simulink model "PD_Ops"  (R2017a)
settings: Solver=ode15s  StartTime=0.0  StopTime=10  RelTol=1e-4
values from neighbouring files (symbols this model uses):
  Kd = 50*eye(7)    [forwardDynamics.m]
  Kp = 500*eye(7)    [forwardDynamics.m]
  m = num2cell(m)    [CoriolisTerm.m]    (also in GravityTerm.m; InvDynNum.m; InverseDynamics.m = [mA mB mC mD mE mF mG]; MassMatrix.m)
libraries: mblibv1 x36, simulink x2
(part 1 of 2)
settings Model: Creator=litianyi  LastModifiedBy=nathaliemajcherczyk
settings SolverCC: ZeroCrossControl=DisableAll

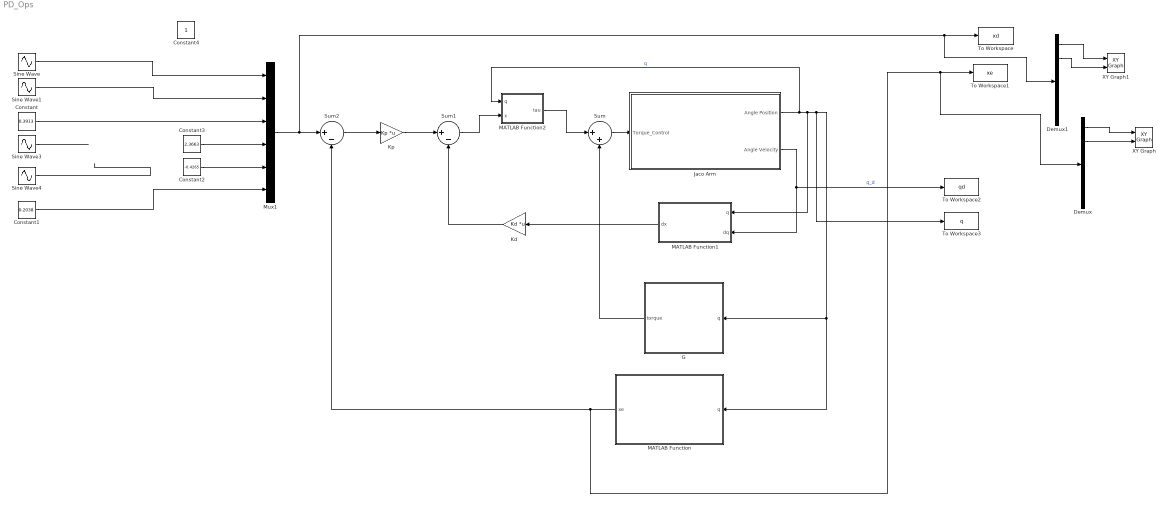
== system PD_Ops ==
  Constant : Constant  Value=0.3913  VectorParams1D=off
  Constant1 : Constant  Value=0.2038  VectorParams1D=off
  Constant2 : Constant  Value=-0.4265  VectorParams1D=off
  Constant3 : Constant  Value=2.3663  VectorParams1D=off
  Constant4 : Constant  VectorParams1D=off
  Demux : Demux  Outputs=6
  Demux1 : Demux  Outputs=6
  G : MATLAB Function  TreatAsAtomicUnit=on
  "Jaco Arm " : Subsystem
  Kd : Gain  Gain=Kd  Multiplication=Matrix(K*u)
  Kp : Gain  Gain=Kp  Multiplication=Matrix(K*u)
  MATLAB Function : MATLAB Function  TreatAsAtomicUnit=on
  MATLAB Function1 : MATLAB Function  TreatAsAtomicUnit=on
  MATLAB Function2 : MATLAB Function  TreatAsAtomicUnit=on
  Mux1 : Mux  Inputs=6
  Sine Wave : Sin  Amplitude=0.2  Bias=0.0075  Phase=pi/2  SampleTime=0
  Sine Wave1 : Sin  Amplitude=0.2  Bias=-0.0204  SampleTime=0
  Sine Wave3 : Sin  Amplitude=10  Phase=pi  SampleTime=0
  Sine Wave4 : Sin  Amplitude=10  Bias=-10  Phase=pi/2  SampleTime=0
  Sum : Sum  Inputs=|++
  Sum1 : Sum  Inputs=|+-
  Sum2 : Sum  Inputs=|+-
  To Workspace : ToWorkspace  VariableName=xd  SaveFormat=Timeseries  SampleTime=-1
  To Workspace1 : ToWorkspace  VariableName=xe  SaveFormat=Timeseries  SampleTime=-1
  To Workspace2 : ToWorkspace  VariableName=qd  SaveFormat=Timeseries  SampleTime=-1
  To Workspace3 : ToWorkspace  VariableName=q  SaveFormat=Timeseries  SampleTime=-1
  XY Graph : simulink/Sinks/XY Graph  xmin=-1  xmax=1  ymin=-1  ymax=1  st=-1
  XY Graph1 : simulink/Sinks/XY Graph  xmin=-1  xmax=1  ymin=-1  ymax=1  st=-1
  wires:
  Kd/1 -> Sum1/2
  "Jaco Arm "/2(Angle Velocity) -> To Workspace2/1, MATLAB Function1/2(dq)  "q_d"
  Kp/1 -> Sum1/1
  "Jaco Arm "/1("Angle Position ") -> MATLAB Function2/1(q), MATLAB Function1/1(q), To Workspace3/1, G/1(q), MATLAB Function/1(q)  "q"
  Sum/1 -> "Jaco Arm "/1("Torque_Control ")
  Sum2/1 -> Kp/1
  G/1(torque) -> Sum/2
  Constant/1 -> Mux1/3
  Constant1/1 -> Mux1/6
  MATLAB Function1/1(dx) -> Kd/1
  MATLAB Function2/1(tau) -> Sum/1
  MATLAB Function/1(xe) -> Demux/1, To Workspace1/1, Sum2/2
  Sum1/1 -> MATLAB Function2/2(x)
  Sine Wave4/1 -> ?
  Sine Wave3/1 -> ?
  Mux1/1 -> Demux1/1, To Workspace/1, Sum2/1
  Demux/1 -> XY Graph/1
  Demux/2 -> XY Graph/2
  Demux1/1 -> XY Graph1/1
  Demux1/2 -> XY Graph1/2
  Sine Wave1/1 -> Mux1/2
  Sine Wave/1 -> Mux1/1
  Constant3/1 -> Mux1/4
  Constant2/1 -> Mux1/5

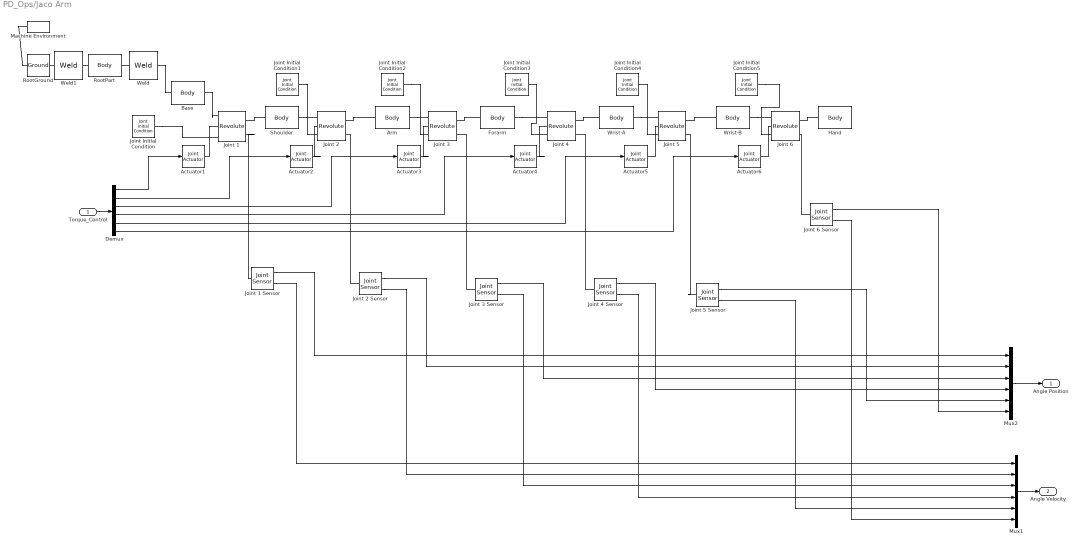
== system PD_Ops/Jaco Arm  ==
  "Torque_Control " : Inport
  Actuator{1..6} (6 alike) : mblibv1/Sensors &  Actuators/Joint Actuator  UpdateFromCAD=off  PhysicalDomain=Mechanical  PortType=blob  ActuationStyle=Force  AngleUnits=deg  ArcVelocityUnits=deg/s  ArcAccelerationUnits=deg/s^2  CoordPositionUnits=m  VelocityUnits=m/s  AccelerationUnits=m/s^2  ForceUnits=N  TorqueUnits=N-m  ActiveIO=on  Width=1  DialogClass=MechanicalActuatorBlock  Primitive=R1  ReferenceFrame=Absolute (World)
      settings: SourceProductName=Simscape Multibody  SourceProductBaseCode=MS
  Arm : mblibv1/Bodies/Body  LConnTagsString=CS2  RConnTagsString=CS3  UpdateFromCAD=on  DialogClass=MechanicalBodyBlock  Mass=1.056  MassUnits=kg  InertiaUnits=kg*m^2  Inertia=[0.0375645,-1.33324e-07,0.000108785;-1.33324e-07,0.0372402,-2.39225e-07;0.000108785,-2.39225e-07,0.00059301]  Shape=Cylinder  ShapeDims=[1 1]  ShapeUnits=m  ShapeUse=false  Density=1  DensityUnits=kg/m^3  DensityUse=false  GraphicsMode=GFXFILE  GraphicsFileName=Jaco_3_7 - arm_ass-1.STL  BodyColorSelMode=COLORPALETTE  BodyColor=[0.752941;0.752941;0.752941]  AttachedToCS=CS1  CG=Right$CG$[0.10282 0.0944444 0.508793]$WORLD$WORLD$m$[0.695251 0.715707 -0.0662524;0.718767 -0.692291 0.0640847;0 -0.092175 -0.995743]$3x3 Transform$rad$WORLD$false$none  WorkingFrames=Right$CS1$[-0.183907 0.105598 0.903425]$WORLD$WORLD$m$[0.695251 0.715707 -0.0662524;0.718767 -0.692291 0.0640847;0 -0.092175 -0.995743]$3x3 Transform$rad$WORLD$false$none#Left$CS2$[0.0767642 0.095252 0.300589]$WORLD$WORLD$m$[1 0 0;0 1 0;0 0 1]$3x3 Transform$rad$WORLD$true$none#Right$CS3$[0.10358 0.0686179 0.708843]$WORLD$WORLD$m$[1 0 0;0 1 0;0 0 1]$3x3 Transform$rad$WORLD$true$none  CGPos=[0.10282 0.0944444 0.508793]  CGRot=[0.695251 0.715707 -0.0662524;0.718767 -0.692291 0.0640847;0 -0.092175 -0.995743]  CS0Pos=[]  CS0Rot=[]  CS1Pos=[-0.183907 0.105598 0.903425]  CS1Rot=[0.695251 0.715707 -0.0662524;0.718767 -0.692291 0.0640847;0 -0.092175 -0.995743]  CS2Pos=[0.0767642 0.095252 0.300589]  CS2Rot=[1 0 0;0 1 0;0 0 1]  CS3Pos=[0.10358 0.0686179 0.708843]  CS3Rot=[1 0 0;0 1 0;0 0 1]  CS4Pos=[]  CS4Rot=[]  CS5Pos=[]  CS5Rot=[]  CS6Pos=[]  CS6Rot=[]  CS7Pos=[]  CS7Rot=[]  CS8Pos=[]  CS8Rot=[]  CS9Pos=[]  CS9Rot=[]  CS10Pos=[]  CS10Rot=[]  CS11Pos=[]  CS11Rot=[]  CS12Pos=[]  CS12Rot=[]  CS13Pos=[]  CS13Rot=[]  CS14Pos=[]  CS14Rot=[]  CS15Pos=[]  CS15Rot=[]  CS16Pos=[]  CS16Rot=[]  CS17Pos=[]  CS17Rot=[]  CS18Pos=[]  CS18Rot=[]  CS19Pos=[]  CS19Rot=[]  CS20Pos=[]  CS20Rot=[]
      settings: SourceProductName=Simscape Multibody  SourceProductBaseCode=MS
  Base : mblibv1/Bodies/Body  LConnTagsString=CS2  RConnTagsString=CS3  UpdateFromCAD=on  DialogClass=MechanicalBodyBlock  Mass=0.570939  MassUnits=kg  InertiaUnits=kg*m^2  Inertia=[0.00175947,1.92772e-07,-3.1782e-05;1.92772e-07,0.00176256,-3.18122e-05;-3.1782e-05,-3.18122e-05,0.000478232]  Shape=Cylinder  ShapeDims=[1 1]  ShapeUnits=m  ShapeUse=false  Density=1  DensityUnits=kg/m^3  DensityUse=false  GraphicsMode=GFXFILE  GraphicsFileName=Jaco_3_7 - base_ass-1.STL  BodyColorSelMode=COLORPALETTE  BodyColor=[0.752941;0.752941;0.752941]  AttachedToCS=CS1  CG=Right$CG$[0.0747134 0.093124 0.128067]$WORLD$WORLD$m$[1 0 0;0 1 0;0 0 1]$3x3 Transform$rad$WORLD$false$none  WorkingFrames=Right$CS1$[0.106448 0.0299726 -0.0762042]$WORLD$WORLD$m$[1 0 0;0 1 0;0 0 1]$3x3 Transform$rad$WORLD$false$none#Left$CS2$[0.0747134 0.093124 0.128067]$WORLD$WORLD$m$[1 0 0;0 1 0;0 0 1]$3x3 Transform$rad$WORLD$true$none#Right$CS3$[0.0753736 0.0938145 0.182089]$WORLD$WORLD$m$[1 0 0;0 1 0;0 0 1]$3x3 Transform$rad$WORLD$true$none  CGPos=[0.0747134 0.093124 0.128067]  CGRot=[1 0 0;0 1 0;0 0 1]  CS0Pos=[]  CS0Rot=[]  CS1Pos=[0.106448 0.0299726 -0.0762042]  CS1Rot=[1 0 0;0 1 0;0 0 1]  CS2Pos=[0.0747134 0.093124 0.128067]  CS2Rot=[1 0 0;0 1 0;0 0 1]  CS3Pos=[0.0753736 0.0938145 0.182089]  CS3Rot=[1 0 0;0 1 0;0 0 1]  CS4Pos=[]  CS4Rot=[]  CS5Pos=[]  CS5Rot=[]  CS6Pos=[]  CS6Rot=[]  CS7Pos=[]  CS7Rot=[]  CS8Pos=[]  CS8Rot=[]  CS9Pos=[]  CS9Rot=[]  CS10Pos=[]  CS10Rot=[]  CS11Pos=[]  CS11Rot=[]  CS12Pos=[]  CS12Rot=[]  CS13Pos=[]  CS13Rot=[]  CS14Pos=[]  CS14Rot=[]  CS15Pos=[]  CS15Rot=[]  CS16Pos=[]  CS16Rot=[]  CS17Pos=[]  CS17Rot=[]  CS18Pos=[]  CS18Rot=[]  CS19Pos=[]  CS19Rot=[]  CS20Pos=[]  CS20Rot=[]
      settings: SourceProductName=Simscape Multibody  SourceProductBaseCode=MS
  Demux : Demux  Outputs=6
  Forarm : mblibv1/Bodies/Body  LConnTagsString=CS2  RConnTagsString=CS3  UpdateFromCAD=on  DialogClass=MechanicalBodyBlock  Mass=0.735414  MassUnits=kg  InertiaUnits=kg*m^2  Inertia=[0.00626271,-0.000115651,1.81814e-08;-0.000115651,0.000377159,4.13244e-07;1.81814e-08,4.13244e-07,0.00610747]  Shape=Cylinder  ShapeDims=[1 1]  ShapeUnits=m  ShapeUse=false  Density=1  DensityUnits=kg/m^3  DensityUse=false  GraphicsMode=GFXFILE  GraphicsFileName=Jaco_3_7 - forarm_ass-1.STL  BodyColorSelMode=COLORPALETTE  BodyColor=[0.752941;0.752941;0.752941]  AttachedToCS=CS1  CG=Right$CG$[0.142291 0.0111153 0.740623]$WORLD$WORLD$m$[0.695251 0.650811 0.305076;0.718767 -0.629518 -0.295094;0 0.424443 -0.905455]$3x3 Transform$rad$WORLD$false$none  WorkingFrames=Right$CS1$[-0.0310579 0.0970807 0.899014]$WORLD$WORLD$m$[0.695251 0.650811 0.305076;0.718767 -0.629518 -0.295094;0 0.424443 -0.905455]$3x3 Transform$rad$WORLD$false$none#Left$CS2$[0.10358 0.0686179 0.708843]$WORLD$WORLD$m$[1 0 0;0 1 0;0 0 1]$3x3 Transform$rad$WORLD$true$none#Right$CS3$[0.230802 -0.0700932 0.796915]$WORLD$WORLD$m$[1 0 0;0 1 0;0 0 1]$3x3 Transform$rad$WORLD$true$none  CGPos=[0.142291 0.0111153 0.740623]  CGRot=[0.695251 0.650811 0.305076;0.718767 -0.629518 -0.295094;0 0.424443 -0.905455]  CS0Pos=[]  CS0Rot=[]  CS1Pos=[-0.0310579 0.0970807 0.899014]  CS1Rot=[0.695251 0.650811 0.305076;0.718767 -0.629518 -0.295094;0 0.424443 -0.905455]  CS2Pos=[0.10358 0.0686179 0.708843]  CS2Rot=[1 0 0;0 1 0;0 0 1]  CS3Pos=[0.230802 -0.0700932 0.796915]  CS3Rot=[1 0 0;0 1 0;0 0 1]  CS4Pos=[]  CS4Rot=[]  CS5Pos=[]  CS5Rot=[]  CS6Pos=[]  CS6Rot=[]  CS7Pos=[]  CS7Rot=[]  CS8Pos=[]  CS8Rot=[]  CS9Pos=[]  CS9Rot=[]  CS10Pos=[]  CS10Rot=[]  CS11Pos=[]  CS11Rot=[]  CS12Pos=[]  CS12Rot=[]  CS13Pos=[]  CS13Rot=[]  CS14Pos=[]  CS14Rot=[]  CS15Pos=[]  CS15Rot=[]  CS16Pos=[]  CS16Rot=[]  CS17Pos=[]  CS17Rot=[]  CS18Pos=[]  CS18Rot=[]  CS19Pos=[]  CS19Rot=[]  CS20Pos=[]  CS20Rot=[]
      settings: SourceProductName=Simscape Multibody  SourceProductBaseCode=MS
  Hand : mblibv1/Bodies/Body  LConnTagsString=CS2  UpdateFromCAD=on  DialogClass=MechanicalBodyBlock  Mass=0.395999  MassUnits=kg  InertiaUnits=kg*m^2  Inertia=[0.00124769,-0.000197969,-5.51354e-06;-0.000197969,0.000409818,-2.12169e-05;-5.51354e-06,-2.12169e-05,0.00139509]  Shape=Cylinder  ShapeDims=[1 1]  ShapeUnits=m  ShapeUse=false  Density=1  DensityUnits=kg/m^3  DensityUse=false  GraphicsMode=GFXFILE  GraphicsFileName=Jaco_3_7 - Hand_ass-1.STL  BodyColorSelMode=COLORPALETTE  BodyColor=[0.752941;0.752941;0.752941]  AttachedToCS=CS1  CG=Right$CG$[0.35442 -0.232757 0.799495]$WORLD$WORLD$m$[-0.439555 0.858973 -0.262597;-0.828489 -0.500657 -0.250895;-0.346983 0.107276 0.931716]$3x3 Transform$rad$WORLD$false$none  WorkingFrames=Right$CS1$[0.362295 -0.115327 0.65151]$WORLD$WORLD$m$[-0.439555 0.858973 -0.262597;-0.828489 -0.500657 -0.250895;-0.346983 0.107276 0.931716]$3x3 Transform$rad$WORLD$false$none#Left$CS2$[0.306767 -0.196631 0.795235]$WORLD$WORLD$m$[1 0 0;0 1 0;0 0 1]$3x3 Transform$rad$WORLD$true$none  CGPos=[0.35442 -0.232757 0.799495]  CGRot=[-0.439555 0.858973 -0.262597;-0.828489 -0.500657 -0.250895;-0.346983 0.107276 0.931716]  CS0Pos=[]  CS0Rot=[]  CS1Pos=[0.362295 -0.115327 0.65151]  CS1Rot=[-0.439555 0.858973 -0.262597;-0.828489 -0.500657 -0.250895;-0.346983 0.107276 0.931716]  CS2Pos=[0.306767 -0.196631 0.795235]  CS2Rot=[1 0 0;0 1 0;0 0 1]  CS3Pos=[]  CS3Rot=[]  CS4Pos=[]  CS4Rot=[]  CS5Pos=[]  CS5Rot=[]  CS6Pos=[]  CS6Rot=[]  CS7Pos=[]  CS7Rot=[]  CS8Pos=[]  CS8Rot=[]  CS9Pos=[]  CS9Rot=[]  CS10Pos=[]  CS10Rot=[]  CS11Pos=[]  CS11Rot=[]  CS12Pos=[]  CS12Rot=[]  CS13Pos=[]  CS13Rot=[]  CS14Pos=[]  CS14Rot=[]  CS15Pos=[]  CS15Rot=[]  CS16Pos=[]  CS16Rot=[]  CS17Pos=[]  CS17Rot=[]  CS18Pos=[]  CS18Rot=[]  CS19Pos=[]  CS19Rot=[]  CS20Pos=[]  CS20Rot=[]
      settings: SourceProductName=Simscape Multibody  SourceProductBaseCode=MS
  Joint 1 : mblibv1/Joints/Revolute  LConnTagsString=__newl0|SA1|SA2  RConnTagsString=__newr0|SA1  UpdateFromCAD=on  NumSAPorts=3  CutJoint=off  MarkAsCut=off  Primitives=prismatic  PrimitiveProps=R1$World$[0,0,1]$revolute  DialogClass=JointBlock  R1Axis=[0,0,1]
      settings: SourceProductName=Simscape Multibody  SourceProductBaseCode=MS
  Joint 1 Sensor : mblibv1/Sensors &  Actuators/Joint Sensor  UpdateFromCAD=off  PhysicalDomain=Mechanical  PortType=blob  Muxed=off  Pose=off  Angle=on  AngleUnits=rad  ArcVelocity=on  ArcVelocityUnits=rad/s  ArcAcceleration=off  ArcAccelerationUnits=deg/s^2  CoordPosition=on  CoordPositionUnits=m  Velocity=off  VelocityUnits=m/s  Acceleration=off  AccelerationUnits=m/s^2  Quaternion=on  QuaternionDT=off  QuaternionDDT=off  QuaternionUnits=off  OutputVector=[1]  ActiveIO=on  Width=2  DialogClass=MechanicalSensorBlock  Primitive=R1  Force=off  ForceUnits=N  Torque=off  TorqueUnits=N*m  ReferenceFrame=Absolute (World)  ReactionSensedSide=Base  ReactionReferenceFrame=Absolute (World)  ReactionForce=off  ReactionForceUnits=N  ReactionMoment=off  ReactionMomentUnits=N*m
      settings: SourceProductName=Simscape Multibody  SourceProductBaseCode=MS
  Joint 2 : mblibv1/Joints/Revolute  LConnTagsString=__newl0|SA1|SA2  RConnTagsString=__newr0|SA1  UpdateFromCAD=on  NumSAPorts=3  CutJoint=off  MarkAsCut=off  Primitives=prismatic  PrimitiveProps=R1$World$[0.695251,0.718767,0]$revolute  DialogClass=JointBlock  R1Axis=[0.695251,0.718767,0]
      settings: SourceProductName=Simscape Multibody  SourceProductBaseCode=MS
  Joint 2 Sensor : mblibv1/Sensors &  Actuators/Joint Sensor  UpdateFromCAD=off  PhysicalDomain=Mechanical  PortType=blob  Muxed=off  Pose=off  Angle=on  AngleUnits=rad  ArcVelocity=on  ArcVelocityUnits=rad/s  ArcAcceleration=off  ArcAccelerationUnits=deg/s^2  CoordPosition=on  CoordPositionUnits=m  Velocity=off  VelocityUnits=m/s  Acceleration=off  AccelerationUnits=m/s^2  Quaternion=on  QuaternionDT=off  QuaternionDDT=off  QuaternionUnits=off  OutputVector=[1]  ActiveIO=on  Width=2  DialogClass=MechanicalSensorBlock  Primitive=R1  Force=off  ForceUnits=N  Torque=off  TorqueUnits=N*m  ReferenceFrame=Absolute (World)  ReactionSensedSide=Base  ReactionReferenceFrame=Absolute (World)  ReactionForce=off  ReactionForceUnits=N  ReactionMoment=off  ReactionMomentUnits=N*m
      settings: SourceProductName=Simscape Multibody  SourceProductBaseCode=MS
  Joint 3 : mblibv1/Joints/Revolute  LConnTagsString=__newl0|SA1|SA2  RConnTagsString=__newr0|SA1  UpdateFromCAD=on  NumSAPorts=3  CutJoint=off  MarkAsCut=off  Primitives=prismatic  PrimitiveProps=R1$World$[-0.695251,-0.718767,0]$revolute  DialogClass=JointBlock  R1Axis=[-0.695251,-0.718767,0]
      settings: SourceProductName=Simscape Multibody  SourceProductBaseCode=MS
  Joint 3 Sensor : mblibv1/Sensors &  Actuators/Joint Sensor  UpdateFromCAD=off  PhysicalDomain=Mechanical  PortType=blob  Muxed=off  Pose=off  Angle=on  AngleUnits=rad  ArcVelocity=on  ArcVelocityUnits=rad/s  ArcAcceleration=off  ArcAccelerationUnits=deg/s^2  CoordPosition=on  CoordPositionUnits=m  Velocity=off  VelocityUnits=m/s  Acceleration=off  AccelerationUnits=m/s^2  Quaternion=on  QuaternionDT=off  QuaternionDDT=off  QuaternionUnits=off  OutputVector=[1]  ActiveIO=on  Width=2  DialogClass=MechanicalSensorBlock  Primitive=R1  Force=off  ForceUnits=N  Torque=off  TorqueUnits=N*m  ReferenceFrame=Absolute (World)  ReactionSensedSide=Base  ReactionReferenceFrame=Absolute (World)  ReactionForce=off  ReactionForceUnits=N  ReactionMoment=off  ReactionMomentUnits=N*m
      settings: SourceProductName=Simscape Multibody  SourceProductBaseCode=MS
  Joint 4 : mblibv1/Joints/Revolute  LConnTagsString=__newl0|SA1|SA2  RConnTagsString=__newr0|SA1  UpdateFromCAD=on  NumSAPorts=3  CutJoint=off  MarkAsCut=off  Primitives=prismatic  PrimitiveProps=R1$World$[0.650811,-0.629518,0.424443]$revolute  DialogClass=JointBlock  R1Axis=[0.650811,-0.629518,0.424443]
      settings: SourceProductName=Simscape Multibody  SourceProductBaseCode=MS
  Joint 4 Sensor : mblibv1/Sensors &  Actuators/Joint Sensor  UpdateFromCAD=off  PhysicalDomain=Mechanical  PortType=blob  Muxed=off  Pose=off  Angle=on  AngleUnits=rad  ArcVelocity=on  ArcVelocityUnits=rad/s  ArcAcceleration=off  ArcAccelerationUnits=deg/s^2  CoordPosition=on  CoordPositionUnits=m  Velocity=off  VelocityUnits=m/s  Acceleration=off  AccelerationUnits=m/s^2  Quaternion=on  QuaternionDT=off  QuaternionDDT=off  QuaternionUnits=off  OutputVector=[1]  ActiveIO=on  Width=2  DialogClass=MechanicalSensorBlock  Primitive=R1  Force=off  ForceUnits=N  Torque=off  TorqueUnits=N*m  ReferenceFrame=Absolute (World)  ReactionSensedSide=Base  ReactionReferenceFrame=Absolute (World)  ReactionForce=off  ReactionForceUnits=N  ReactionMoment=off  ReactionMomentUnits=N*m
      settings: SourceProductName=Simscape Multibody  SourceProductBaseCode=MS
  Joint 5 : mblibv1/Joints/Revolute  LConnTagsString=__newl0|SA1|SA2  RConnTagsString=__newr0|SA1  UpdateFromCAD=on  NumSAPorts=3  CutJoint=off  MarkAsCut=off  Primitives=prismatic  PrimitiveProps=R1$World$[0.15169,-0.946456,-0.284976]$revolute  DialogClass=JointBlock  R1Axis=[0.15169,-0.946456,-0.284976]
      settings: SourceProductName=Simscape Multibody  SourceProductBaseCode=MS
  Joint 5 Sensor : mblibv1/Sensors &  Actuators/Joint Sensor  UpdateFromCAD=off  PhysicalDomain=Mechanical  PortType=blob  Muxed=off  Pose=off  Angle=on  AngleUnits=rad  ArcVelocity=on  ArcVelocityUnits=rad/s  ArcAcceleration=off  ArcAccelerationUnits=deg/s^2  CoordPosition=on  CoordPositionUnits=m  Velocity=off  VelocityUnits=m/s  Acceleration=off  AccelerationUnits=m/s^2  Quaternion=on  QuaternionDT=off  QuaternionDDT=off  QuaternionUnits=off  OutputVector=[1]  ActiveIO=on  Width=2  DialogClass=MechanicalSensorBlock  Primitive=R1  Force=off  ForceUnits=N  Torque=off  TorqueUnits=N*m  ReferenceFrame=Absolute (World)  ReactionSensedSide=Base  ReactionReferenceFrame=Absolute (World)  ReactionForce=off  ReactionForceUnits=N  ReactionMoment=off  ReactionMomentUnits=N*m
      settings: SourceProductName=Simscape Multibody  SourceProductBaseCode=MS
  Joint 6 : mblibv1/Joints/Revolute  LConnTagsString=__newl0|SA1|SA2  RConnTagsString=__newr0|SA1  UpdateFromCAD=on  NumSAPorts=3  CutJoint=off  MarkAsCut=off  Primitives=prismatic  PrimitiveProps=R1$World$[0.858973,-0.500657,0.107276]$revolute  DialogClass=JointBlock  R1Axis=[0.858973,-0.500657,0.107276]
      settings: SourceProductName=Simscape Multibody  SourceProductBaseCode=MS
  Joint 6 Sensor : mblibv1/Sensors &  Actuators/Joint Sensor  UpdateFromCAD=off  PhysicalDomain=Mechanical  PortType=blob  Muxed=off  Pose=off  Angle=on  AngleUnits=rad  ArcVelocity=on  ArcVelocityUnits=rad/s  ArcAcceleration=off  ArcAccelerationUnits=deg/s^2  CoordPosition=on  CoordPositionUnits=m  Velocity=off  VelocityUnits=m/s  Acceleration=off  AccelerationUnits=m/s^2  Quaternion=on  QuaternionDT=off  QuaternionDDT=off  QuaternionUnits=off  OutputVector=[1]  ActiveIO=on  Width=2  DialogClass=MechanicalSensorBlock  Primitive=R1  Force=off  ForceUnits=N  Torque=off  TorqueUnits=N*m  ReferenceFrame=Absolute (World)  ReactionSensedSide=Base  ReactionReferenceFrame=Absolute (World)  ReactionForce=off  ReactionForceUnits=N  ReactionMoment=off  ReactionMomentUnits=N*m
      settings: SourceProductName=Simscape Multibody  SourceProductBaseCode=MS
  Joint Initial Condition : mblibv1/Sensors &  Actuators/Joint Initial Condition  UpdateFromCAD=off  LeftPortType=blob  RightPortType=blob  PhysicalDomain=mechanical  DialogClass=InitialConditionBlock  InitialConditions=P1$false$0$m$deg$0$m/s$deg/s#P2$false$0$m$deg$0$m/s$deg/s#P3$false$0$m$deg$0$m/s$deg/s#R1$true$0.81$m$rad$0$m/s$rad/s#R2$false$0$m$deg$0$m/s$deg/s#R3$false$0$m$deg$0$m/s$deg/s#S$false$0$m$deg$0$m/s$deg/s  P1PIC=0  P1VIC=0  P2PIC=0  P2VIC=0  P3PIC=0  P3VIC=0  R1PIC=0.81  R1VIC=0  R2PIC=0  R2VIC=0  R3PIC=0  R3VIC=0  SPIC=0  SVIC=0
      settings: SourceProductName=Simscape Multibody  SourceProductBaseCode=MS
  Joint Initial Condition1 : mblibv1/Sensors &  Actuators/Joint Initial Condition  UpdateFromCAD=off  LeftPortType=blob  RightPortType=blob  PhysicalDomain=mechanical  DialogClass=InitialConditionBlock  InitialConditions=P1$false$0$m$deg$0$m/s$deg/s#P2$false$0$m$deg$0$m/s$deg/s#P3$false$0$m$deg$0$m/s$deg/s#R1$true$-0.6915$m$rad$0$m/s$rad/s#R2$false$0$m$deg$0$m/s$deg/s#R3$false$0$m$deg$0$m/s$deg/s#S$false$0$m$deg$0$m/s$deg/s  P1PIC=0  P1VIC=0  P2PIC=0  P2VIC=0  P3PIC=0  P3VIC=0  R1PIC=-0.6915  R1VIC=0  R2PIC=0  R2VIC=0  R3PIC=0  R3VIC=0  SPIC=0  SVIC=0
      settings: SourceProductName=Simscape Multibody  SourceProductBaseCode=MS
  Joint Initial Condition2 : mblibv1/Sensors &  Actuators/Joint Initial Condition  UpdateFromCAD=off  LeftPortType=blob  RightPortType=blob  PhysicalDomain=mechanical  DialogClass=InitialConditionBlock  InitialConditions=P1$false$0$m$deg$0$m/s$deg/s#P2$false$0$m$deg$0$m/s$deg/s#P3$false$0$m$deg$0$m/s$deg/s#R1$true$1.5708$m$rad$0.2$m/s$rad/s#R2$false$0$m$deg$0$m/s$deg/s#R3$false$0$m$deg$0$m/s$deg/s#S$false$0$m$deg$0$m/s$deg/s  P1PIC=0  P1VIC=0  P2PIC=0  P2VIC=0  P3PIC=0  P3VIC=0  R1PIC=1.5708  R1VIC=0.2  R2PIC=0  R2VIC=0  R3PIC=0  R3VIC=0  SPIC=0  SVIC=0
      settings: SourceProductName=Simscape Multibody  SourceProductBaseCode=MS
  Joint Initial Condition3 : mblibv1/Sensors &  Actuators/Joint Initial Condition  UpdateFromCAD=off  LeftPortType=blob  RightPortType=blob  PhysicalDomain=mechanical  DialogClass=InitialConditionBlock  InitialConditions=P1$false$0$m$deg$0$m/s$deg/s#P2$false$0$m$deg$0$m/s$deg/s#P3$false$0$m$deg$0$m/s$deg/s#R1$true$3.1415$m$rad$0$m/s$rad/s#R2$false$0$m$deg$0$m/s$deg/s#R3$false$0$m$deg$0$m/s$deg/s#S$false$0$m$deg$0$m/s$deg/s  P1PIC=0  P1VIC=0  P2PIC=0  P2VIC=0  P3PIC=0  P3VIC=0  R1PIC=3.1415  R1VIC=0  R2PIC=0  R2VIC=0  R3PIC=0  R3VIC=0  SPIC=0  SVIC=0
      settings: SourceProductName=Simscape Multibody  SourceProductBaseCode=MS
  Joint Initial Condition4 : mblibv1/Sensors &  Actuators/Joint Initial Condition  UpdateFromCAD=off  LeftPortType=blob  RightPortType=blob  PhysicalDomain=mechanical  DialogClass=InitialConditionBlock  InitialConditions=P1$false$0$m$deg$0$m/s$deg/s#P2$false$0$m$deg$0$m/s$deg/s#P3$false$0$m$deg$0$m/s$deg/s#R1$true$-1.70256$m$rad$0$m/s$deg/s#R2$false$0$m$deg$0$m/s$deg/s#R3$false$0$m$deg$0$m/s$deg/s#S$false$0$m$deg$0$m/s$deg/s  P1PIC=0  P1VIC=0  P2PIC=0  P2VIC=0  P3PIC=0  P3VIC=0  R1PIC=-1.70256  R1VIC=0  R2PIC=0  R2VIC=0  R3PIC=0  R3VIC=0  SPIC=0  SVIC=0
      settings: SourceProductName=Simscape Multibody  SourceProductBaseCode=MS
  Joint Initial Condition5 : mblibv1/Sensors &  Actuators/Joint Initial Condition  UpdateFromCAD=off  LeftPortType=blob  RightPortType=blob  PhysicalDomain=mechanical  DialogClass=InitialConditionBlock  InitialConditions=P1$false$0$m$deg$0$m/s$deg/s#P2$false$0$m$deg$0$m/s$deg/s#P3$false$0$m$deg$0$m/s$deg/s#R1$true$0.8222$m$rad$0$m/s$rad/s#R2$false$0$m$deg$0$m/s$deg/s#R3$false$0$m$deg$0$m/s$deg/s#S$false$0$m$deg$0$m/s$deg/s  P1PIC=0  P1VIC=0  P2PIC=0  P2VIC=0  P3PIC=0  P3VIC=0  R1PIC=0.8222  R1VIC=0  R2PIC=0  R2VIC=0  R3PIC=0  R3VIC=0  SPIC=0  SVIC=0
      settings: SourceProductName=Simscape Multibody  SourceProductBaseCode=MS
  Machine Environment : mblibv1/Bodies/Machine Environment  PortType=env  PhysicalDomain=Mechanical  DialogTemplateClass=MECH.MachineEnvironment  SyncWhenCopied=off  Gravity=[0 0 -9.81]  GravityUnits=m/s^2  GravityAsSignal=off  Dimensionality=Auto-detect  AnalysisType=Forward dynamics  LinearAssemblyTolerance=1e-3  LinearAssemblyToleranceUnits=m  AngularAssemblyTolerance=1e-3  AngularAssemblyToleranceUnits=rad  ConstraintSolverType=Stabilizing  ConstraintRelTolerance=1e-4  ConstraintAbsTolerance=1e-4  UseRobustSingularityHandling=off  RedundancyAnalysisToleranceType=Automatically select tolerance  RedundancyAnalysisTolerance=1e-14  StatePerturbationType=Fixed  PerturbationSize=1e-5  VisualizeMachine=on  BodyVisualizationType=Use model default body geometries  BodyColorSelMode=Use model default  DefaultBodyColor=[1 0 0]
      settings: SourceProductName=Simscape Multibody  SourceProductBaseCode=MS
  Mux1 : Mux  Inputs=6
  Mux2 : Mux  Inputs=6
  RootGround : mblibv1/Bodies/Ground  UpdateFromCAD=on  LeftPortType=env  RightPortType=workingframe  PhysicalDomain=Mechanical  DialogClass=GroundBlock  CoordPosition=[0.154743,0.00421299,0.535333]  CoordPositionUnits=m  StateVectorMgrId=1  MachineId=[2 0]  ShowEnvPort=on  ParameterChecksum=[3699419796, 394120427, 2468236942, 3602047536]  TopologyChecksum=[2687420730, 107768908, 3585950869, 4292946198]
      settings: SourceProductName=Simscape Multibody  SourceProductBaseCode=MS
  RootPart : mblibv1/Bodies/Body  LConnTagsString=CS3  RConnTagsString=CS2  UpdateFromCAD=on  DialogClass=MechanicalBodyBlock  Mass=0  MassUnits=kg  InertiaUnits=kg*m^2  Inertia=[0,0,0;0,0,0;0,0,0]  Shape=Cylinder  ShapeDims=[1 1]  ShapeUnits=m  ShapeUse=false  Density=1  DensityUnits=kg/m^3  DensityUse=false  GraphicsMode=MACHINE_DEFAULT  BodyColorSelMode=MACHINE_DEFAULT  BodyColor=[1;0;0]  AttachedToCS=CS1  CG=Right$CG$[0.154743 0.00421299 0.535333]$WORLD$WORLD$m$[1 0 0;0 1 0;0 0 1]$3x3 Transform$rad$WORLD$false$none  WorkingFrames=Right$CS1$[0 0 0]$WORLD$WORLD$m$[1 0 0;0 1 0;0 0 1]$3x3 Transform$rad$WORLD$false$none#Right$CS2$[0.0747134 0.093124 0.128067]$WORLD$WORLD$m$[1 0 0;0 1 0;0 0 1]$3x3 Transform$rad$WORLD$true$none#Left$CS3$[0.154743 0.00421299 0.535333]$WORLD$WORLD$m$[1 0 0;0 1 0;0 0 1]$3x3 Transform$rad$WORLD$true$none  CGPos=[0.154743 0.00421299 0.535333]  CGRot=[1 0 0;0 1 0;0 0 1]  CS0Pos=[]  CS0Rot=[]  CS1Pos=[0 0 0]  CS1Rot=[1 0 0;0 1 0;0 0 1]  CS2Pos=[0.0747134 0.093124 0.128067]  CS2Rot=[1 0 0;0 1 0;0 0 1]  CS3Pos=[0.154743 0.00421299 0.535333]  CS3Rot=[1 0 0;0 1 0;0 0 1]  CS4Pos=[]  CS4Rot=[]  CS5Pos=[]  CS5Rot=[]  CS6Pos=[]  CS6Rot=[]  CS7Pos=[]  CS7Rot=[]  CS8Pos=[]  CS8Rot=[]  CS9Pos=[]  CS9Rot=[]  CS10Pos=[]  CS10Rot=[]  CS11Pos=[]  CS11Rot=[]  CS12Pos=[]  CS12Rot=[]  CS13Pos=[]  CS13Rot=[]  CS14Pos=[]  CS14Rot=[]  CS15Pos=[]  CS15Rot=[]  CS16Pos=[]  CS16Rot=[]  CS17Pos=[]  CS17Rot=[]  CS18Pos=[]  CS18Rot=[]  CS19Pos=[]  CS19Rot=[]  CS20Pos=[]  CS20Rot=[]
      settings: SourceProductName=Simscape Multibody  SourceProductBaseCode=MS
  Shoulder : mblibv1/Bodies/Body  LConnTagsString=CS3  RConnTagsString=CS2  UpdateFromCAD=on  DialogClass=MechanicalBodyBlock  Mass=0.813994  MassUnits=kg  InertiaUnits=kg*m^2  Inertia=[0.0026546,0.000304923,5.38935e-08;0.000304923,0.000595598,-3.17242e-07;5.38935e-08,-3.17242e-07,0.00258406]  Shape=Cylinder  ShapeDims=[1 1]  ShapeUnits=m  ShapeUse=false  Density=1  DensityUnits=kg/m^3  DensityUse=false  GraphicsMode=GFXFILE  GraphicsFileName=Jaco_3_7 - shoulder_ass-1.STL  BodyColorSelMode=COLORPALETTE  BodyColor=[0.752941;0.752941;0.752941]  AttachedToCS=CS1  CG=Right$CG$[0.0698164 0.0880634 0.250193]$WORLD$WORLD$m$[0.695251 0 0.718767;0.718767 0 -0.695251;0 1 0]$3x3 Transform$rad$WORLD$false$none  WorkingFrames=Right$CS1$[-0.0564522 0.142463 0.184725]$WORLD$WORLD$m$[0.695251 0 0.718767;0.718767 0 -0.695251;0 1 0]$3x3 Transform$rad$WORLD$false$none#Right$CS2$[0.0767642 0.095252 0.300589]$WORLD$WORLD$m$[1 0 0;0 1 0;0 0 1]$3x3 Transform$rad$WORLD$true$none#Left$CS3$[0.0753736 0.0938145 0.182089]$WORLD$WORLD$m$[1 0 0;0 1 0;0 0 1]$3x3 Transform$rad$WORLD$true$none  CGPos=[0.0698164 0.0880634 0.250193]  CGRot=[0.695251 0 0.718767;0.718767 0 -0.695251;0 1 0]  CS0Pos=[]  CS0Rot=[]  CS1Pos=[-0.0564522 0.142463 0.184725]  CS1Rot=[0.695251 0 0.718767;0.718767 0 -0.695251;0 1 0]  CS2Pos=[0.0767642 0.095252 0.300589]  CS2Rot=[1 0 0;0 1 0;0 0 1]  CS3Pos=[0.0753736 0.0938145 0.182089]  CS3Rot=[1 0 0;0 1 0;0 0 1]  CS4Pos=[]  CS4Rot=[]  CS5Pos=[]  CS5Rot=[]  CS6Pos=[]  CS6Rot=[]  CS7Pos=[]  CS7Rot=[]  CS8Pos=[]  CS8Rot=[]  CS9Pos=[]  CS9Rot=[]  CS10Pos=[]  CS10Rot=[]  CS11Pos=[]  CS11Rot=[]  CS12Pos=[]  CS12Rot=[]  CS13Pos=[]  CS13Rot=[]  CS14Pos=[]  CS14Rot=[]  CS15Pos=[]  CS15Rot=[]  CS16Pos=[]  CS16Rot=[]  CS17Pos=[]  CS17Rot=[]  CS18Pos=[]  CS18Rot=[]  CS19Pos=[]  CS19Rot=[]  CS20Pos=[]  CS20Rot=[]
      settings: SourceProductName=Simscape Multibody  SourceProductBaseCode=MS
  Weld : mblibv1/Joints/Weld  LConnTagsString=__newl0  RConnTagsString=__newr0  UpdateFromCAD=on  NumSAPorts=0  CutJoint=off  MarkAsCut=off  Primitives=weld  PrimitiveProps=W$WORLD$[0.57735,0.57735,0.57735]$weld  DialogClass=JointBlock  WAxis=[0.57735,0.57735,0.57735]
      settings: SourceProductName=Simscape Multibody  SourceProductBaseCode=MS
  Weld1 : mblibv1/Joints/Weld  LConnTagsString=__newl0  RConnTagsString=__newr0  UpdateFromCAD=on  NumSAPorts=0  CutJoint=off  MarkAsCut=off  Primitives=weld  PrimitiveProps=W$WORLD$[0.57735,0.57735,0.57735]$weld  DialogClass=JointBlock  WAxis=[0.57735,0.57735,0.57735]
      settings: SourceProductName=Simscape Multibody  SourceProductBaseCode=MS
  Wrist-A : mblibv1/Bodies/Body  LConnTagsString=CS3  RConnTagsString=CS2  UpdateFromCAD=on  DialogClass=MechanicalBodyBlock  Mass=0.44698  MassUnits=kg  InertiaUnits=kg*m^2  Inertia=[0.000407036,-3.06246e-08,5.0605e-09;-3.06246e-08,0.000239744,-8.7175e-05;5.0605e-09,-8.7175e-05,0.000376656]  Shape=Cylinder  ShapeDims=[1 1]  ShapeUnits=m  ShapeUse=false  Density=1  DensityUnits=kg/m^3  DensityUse=false  GraphicsMode=GFXFILE  GraphicsFileName=Jaco_3_7 - wrist1_ass-1.STL  BodyColorSelMode=COLORPALETTE  BodyColor=[0.752941;0.752941;0.752941]  AttachedToCS=CS1  CG=Right$CG$[0.251866 -0.101707 0.805258]$WORLD$WORLD$m$[0.709409 0.650811 -0.270524;0.30501 -0.629518 -0.714616;-0.63538 0.424443 -0.64509]$3x3 Transform$rad$WORLD$false$none  WorkingFrames=Right$CS1$[0.228148 -0.0304193 0.852839]$WORLD$WORLD$m$[0.709409 0.650811 -0.270524;0.30501 -0.629518 -0.714616;-0.63538 0.424443 -0.64509]$3x3 Transform$rad$WORLD$false$none#Right$CS2$[0.264276 -0.136155 0.802577]$WORLD$WORLD$m$[1 0 0;0 1 0;0 0 1]$3x3 Transform$rad$WORLD$true$none#Left$CS3$[0.230802 -0.0700932 0.796915]$WORLD$WORLD$m$[1 0 0;0 1 0;0 0 1]$3x3 Transform$rad$WORLD$true$none  CGPos=[0.251866 -0.101707 0.805258]  CGRot=[0.709409 0.650811 -0.270524;0.30501 -0.629518 -0.714616;-0.63538 0.424443 -0.64509]  CS0Pos=[]  CS0Rot=[]  CS1Pos=[0.228148 -0.0304193 0.852839]  CS1Rot=[0.709409 0.650811 -0.270524;0.30501 -0.629518 -0.714616;-0.63538 0.424443 -0.64509]  CS2Pos=[0.264276 -0.136155 0.802577]  CS2Rot=[1 0 0;0 1 0;0 0 1]  CS3Pos=[0.230802 -0.0700932 0.796915]  CS3Rot=[1 0 0;0 1 0;0 0 1]  CS4Pos=[]  CS4Rot=[]  CS5Pos=[]  CS5Rot=[]  CS6Pos=[]  CS6Rot=[]  CS7Pos=[]  CS7Rot=[]  CS8Pos=[]  CS8Rot=[]  CS9Pos=[]  CS9Rot=[]  CS10Pos=[]  CS10Rot=[]  CS11Pos=[]  CS11Rot=[]  CS12Pos=[]  CS12Rot=[]  CS13Pos=[]  CS13Rot=[]  CS14Pos=[]  CS14Rot=[]  CS15Pos=[]  CS15Rot=[]  CS16Pos=[]  CS16Rot=[]  CS17Pos=[]  CS17Rot=[]  CS18Pos=[]  CS18Rot=[]  CS19Pos=[]  CS19Rot=[]  CS20Pos=[]  CS20Rot=[]
      settings: SourceProductName=Simscape Multibody  SourceProductBaseCode=MS
  Wrist-B : mblibv1/Bodies/Body  LConnTagsString=CS3  RConnTagsString=CS2  UpdateFromCAD=on  DialogClass=MechanicalBodyBlock  Mass=0.44698  MassUnits=kg  InertiaUnits=kg*m^2  Inertia=[0.000407036,-3.06246e-08,5.0605e-09;-3.06246e-08,0.000239744,-8.7175e-05;5.0605e-09,-8.7175e-05,0.000376656]  Shape=Cylinder  ShapeDims=[1 1]  ShapeUnits=m  ShapeUse=false  Density=1  DensityUnits=kg/m^3  DensityUse=false  GraphicsMode=GFXFILE  GraphicsFileName=Jaco_3_7 - wrist2_ass-1.STL  BodyColorSelMode=COLORPALETTE  BodyColor=[0.752941;0.752941;0.752941]  AttachedToCS=CS1  CG=Right$CG$[0.28076 -0.170724 0.795794]$WORLD$WORLD$m$[-0.298122 0.15169 0.942398;-0.318695 -0.946456 0.0515257;0.899754 -0.284976 0.330502]$3x3 Transform$rad$WORLD$false$none  WorkingFrames=Right$CS1$[0.211333 -0.128563 0.759589]$WORLD$WORLD$m$[-0.298122 0.15169 0.942398;-0.318695 -0.946456 0.0515257;0.899754 -0.284976 0.330502]$3x3 Transform$rad$WORLD$false$none#Right$CS2$[0.306767 -0.196631 0.795235]$WORLD$WORLD$m$[1 0 0;0 1 0;0 0 1]$3x3 Transform$rad$WORLD$true$none#Left$CS3$[0.264276 -0.136155 0.802577]$WORLD$WORLD$m$[1 0 0;0 1 0;0 0 1]$3x3 Transform$rad$WORLD$true$none  CGPos=[0.28076 -0.170724 0.795794]  CGRot=[-0.298122 0.15169 0.942398;-0.318695 -0.946456 0.0515257;0.899754 -0.284976 0.330502]  CS0Pos=[]  CS0Rot=[]  CS1Pos=[0.211333 -0.128563 0.759589]  CS1Rot=[-0.298122 0.15169 0.942398;-0.318695 -0.946456 0.0515257;0.899754 -0.284976 0.330502]  CS2Pos=[0.306767 -0.196631 0.795235]  CS2Rot=[1 0 0;0 1 0;0 0 1]  CS3Pos=[0.264276 -0.136155 0.802577]  CS3Rot=[1 0 0;0 1 0;0 0 1]  CS4Pos=[]  CS4Rot=[]  CS5Pos=[]  CS5Rot=[]  CS6Pos=[]  CS6Rot=[]  CS7Pos=[]  CS7Rot=[]  CS8Pos=[]  CS8Rot=[]  CS9Pos=[]  CS9Rot=[]  CS10Pos=[]  CS10Rot=[]  CS11Pos=[]  CS11Rot=[]  CS12Pos=[]  CS12Rot=[]  CS13Pos=[]  CS13Rot=[]  CS14Pos=[]  CS14Rot=[]  CS15Pos=[]  CS15Rot=[]  CS16Pos=[]  CS16Rot=[]  CS17Pos=[]  CS17Rot=[]  CS18Pos=[]  CS18Rot=[]  CS19Pos=[]  CS19Rot=[]  CS20Pos=[]  CS20Rot=[]
      settings: SourceProductName=Simscape Multibody  SourceProductBaseCode=MS
  "Angle Position " : Outport
  Angle Velocity : Outport  Port=2
  wires:
  Demux/2 -> Actuator2/1
  Demux/3 -> Actuator3/1
  Demux/4 -> Actuator4/1
  Demux/5 -> Actuator5/1
  Demux/6 -> Actuator6/1
  Joint 3 Sensor/1 -> Mux2/3
  Joint 6 Sensor/1 -> Mux2/6
  Joint 6 Sensor/2 -> Mux1/6
  Demux/1 -> Actuator1/1
  "Torque_Control "/1 -> Demux/1
  Mux2/1 -> "Angle Position "/1
  Joint 1 Sensor/1 -> Mux2/1
  Joint 2 Sensor/1 -> Mux2/2
  Joint 4 Sensor/1 -> Mux2/4
  Joint 5 Sensor/1 -> Mux2/5
  Mux1/1 -> Angle Velocity/1
  Joint 1 Sensor/2 -> Mux1/1
  Joint 2 Sensor/2 -> Mux1/2
  Joint 3 Sensor/2 -> Mux1/3
  Joint 4 Sensor/2 -> Mux1/4
  Joint 5 Sensor/2 -> Mux1/5
  connections:
  Actuator5/RConn1 -- Joint 5/LConn2
  Shoulder/RConn1 -- Joint 2/LConn1
  Joint 3 Sensor/LConn1 -- Joint 3/RConn2
  Weld/RConn1 -- Base/LConn1
  Joint 3/RConn1 -- Forarm/LConn1
  Joint 5/RConn1 -- Wrist-B/LConn1
  Joint 6/RConn1 -- Hand/LConn1
  Joint 6 Sensor/LConn1 -- Joint 6/RConn2
  Joint 2/RConn1 -- Arm/LConn1
  Actuator3/RConn1 -- Joint 3/LConn2
  Joint 5 Sensor/LConn1 -- Joint 5/RConn2
  Joint 4 Sensor/LConn1 -- Joint 4/RConn2
  Arm/RConn1 -- Joint 3/LConn1
  Actuator6/RConn1 -- Joint 6/LConn2
  Actuator4/RConn1 -- Joint 4/LConn2
  Joint 1/RConn1 -- Shoulder/LConn1
  RootPart/RConn1 -- Weld/LConn1
  Base/RConn1 -- Joint 1/LConn1
  Wrist-A/RConn1 -- Joint 5/LConn1
  Wrist-B/RConn1 -- Joint 6/LConn1
  Weld1/RConn1 -- RootPart/LConn1
  Joint 4/RConn1 -- Wrist-A/LConn1
  Forarm/RConn1 -- Joint 4/LConn1
  Joint 2 Sensor/LConn1 -- Joint 2/RConn2
  RootGround/RConn1 -- Weld1/LConn1
  Actuator2/RConn1 -- Joint 2/LConn2
  Joint 1/LConn2 -- Actuator1/RConn1
  Joint 1/RConn2 -- Joint 1 Sensor/LConn1
  Machine Environment/RConn1 -- RootGround/LConn1
  Joint Initial Condition/RConn1 -- Joint 1/LConn3
  Joint Initial Condition1/RConn1 -- Joint 2/LConn3
  Joint Initial Condition2/RConn1 -- Joint 3/LConn3
  Joint Initial Condition3/RConn1 -- Joint 4/LConn3
  Joint Initial Condition4/RConn1 -- Joint 5/LConn3
  Joint Initial Condition5/RConn1 -- Joint 6/LConn3

== matlab function PD_Ops/MATLAB Function ==
  data: q input; xe output
function xe   = DirectKinematics(q)
% DirectKinematics
%    [ Oe, Re ] = DirectKinematics(q)
%    This function was generated by the Symbolic Math Toolbox version 7.2.
%    23-Apr-2017 13:45:31

q1=q(1);
q2=q(2);
q3=q(3);
q4=q(4);
q5=q(5);
q6=q(6);

t2 = pi.*(1.1e1./3.6e1);
t3 = sin(t2);
t4 = sin(q1);
t5 = cos(q1);
t6 = q2-q3;
t7 = 1.0./t3;
t8 = pi.*(1.1e1./7.2e1);
t9 = sin(t8);
t10 = cos(t2);
t11 = cos(q4);
t12 = t3.*t4.*t11;
t13 = sin(t6);
t14 = cos(t6);
t15 = sin(q4);
t16 = t3.*t5.*t14.*t15;
t34 = t5.*t10.*t13;
t17 = t12+t16-t34;
t18 = cos(q2);
t19 = cos(t8);
t20 = t3.*1.687e3;
t21 = t9.*7.43e2;
t22 = t20+t21;
t23 = t3.*t5.*t11;
t24 = t4.*t10.*t13;
t44 = t3.*t4.*t14.*t15;
t25 = t23+t24-t44;
t26 = sin(q5);
t27 = cos(q3);
t28 = sin(q2);
t29 = sin(q3);
t30 = cos(q5);
t31 = 1.0./t19;
t32 = t19.*4.146e3;
t33 = t32+7.43e2;
t35 = t5.*t11.*t18.*t27;
t36 = t5.*t11.*t28.*t29;
t42 = t4.*t15;
t37 = t35+t36-t42;
t38 = t4.*t10.*t11;
t39 = t3.*t5.*t13;
t40 = t5.*t10.*t14.*t15;
t41 = t38+t39+t40;
t43 = sin(q6);
t45 = t5.*t15;
t46 = t4.*t11.*t18.*t27;
t47 = t4.*t11.*t28.*t29;
t48 = t45+t46+t47;
t49 = t3.*t4.*t13;
t50 = t4.*t10.*t14.*t15;
t53 = t5.*t10.*t11;
t51 = t49+t50-t53;
t52 = cos(q6);
t54 = t10.*t14;
t55 = t3.*t13.*t15;
t56 = t54+t55;
t57 = t3.*t14;
t60 = t10.*t13.*t15;
t58 = t57-t60;
t59 = t3.*t56;
t61 = t10.*t30.*t58;
t70 = t10.*t11.*t13.*t26;
t62 = t59+t61-t70;
t63 = t11.*t13.*t30;
t64 = t3.*t14.*t26;
t71 = t10.*t13.*t15.*t26;
t65 = t63+t64-t71;
t66 = t43.*t65-t52.*t62;
t67 = t10.*t56;
t68 = t3.*t11.*t13.*t26;
t72 = t3.*t30.*t58;
t69 = t67+t68-t72;
xe = [t4.*9.8e-3+t5.*t18.*(4.1e1./1.0e2)-t7.*t22.*(t10.*t17+t3.*t26.*t37+t3.*t30.*t41).*1.0e-4-t7.*t9.*t17.*1.486e-1+t5.*t13.*t31.*t33.*5.0e-5;t5.*(-9.8e-3)+t4.*t18.*(4.1e1./1.0e2)-t7.*t22.*(-t10.*t25+t3.*t26.*t48+t3.*t30.*t51).*1.0e-4+t7.*t9.*t25.*1.486e-1+t4.*t13.*t31.*t33.*5.0e-5;t28.*(4.1e1./1.0e2)-t31.*(-t14+t14.*t19.^2.*2.0+t9.*t13.*t15.*t19.*2.0).*7.43e-2-t14.*t31.*t33.*5.0e-5-t7.*t22.*t69.*1.0e-4+2.755e-1;angle(-t52.*(t26.*t41-t30.*t37)-t52.*(t26.*t51-t30.*t48).*1i-t43.*(-t3.*t17+t10.*t26.*t37+t10.*t30.*t41)-t43.*(t3.*t25+t10.*t26.*t48+t10.*t30.*t51).*1i);angle(t43.*t62.*-1i-t52.*t65.*1i+sqrt(t66.^2+t69.^2));angle(-t67-t68+t72+t43.*t65.*1i-t52.*t62.*1i)];

== matlab function PD_Ops/G ==
  data: q input; torque output
function torque  = gravity(q)
%GRAVITY
%    TORQUE = GRAVITY(Q1,Q2,Q3,Q4,Q5,Q6)

%    This function was generated by the Symbolic Math Toolbox version 5.8.
%    15-Mar-2017 14:16:45

q1=q(1);
q2=q(2);
q3=q(3);
q4=q(4);
q5=q(5);
q6=q(6);

t2 = cos(q2);
t3 = pi.*(1.1e1./3.6e1);
t4 = sin(q3);
t5 = cos(q3);
t6 = sin(q2);
t9 = t2.*t4;
t10 = t5.*t6;
t7 = t9-t10;
t8 = sin(t3);
t11 = 1.0./t8;
t12 = pi.*(1.1e1./7.2e1);
t13 = sin(t12);
t14 = t11.*t13.*(7.43e2./1.0e4);
t15 = cos(t3);
t16 = sin(q4);
t17 = t2.*t5;
t18 = t4.*t6;
t19 = t17+t18;
t20 = sin(q5);
t21 = t7.*t8;
t29 = t15.*t16.*t19;
t22 = t21-t29;
t23 = cos(q4);
t24 = cos(q5);
t25 = cos(q6);
t26 = t7.*t15;
t27 = t8.*t16.*t19;
t28 = t26+t27;
t30 = t20.*t22;
t31 = t19.*t23.*t24;
t32 = t30+t31;
t33 = sin(q6);
t34 = t8.*t28;
t35 = t15.*t22.*t24;
t45 = t15.*t19.*t20.*t23;
t36 = t34+t35-t45;
t37 = t7.*t8.*(2.30993127e8./5.0e9);
t38 = t5.*t6.*(4.1664051e7./7.8125e7);
t39 = t14+2.073e3./1.0e4;
t40 = t14+1.687e3./1.0e4;
t41 = t15.*t28;
t42 = t8.*t19.*t20.*t23;
t43 = t41+t42-t8.*t22.*t24;
t44 = t40.*t43.*(2.033613e6./1.0e5);
t46 = t15.*t28.*(2.1698418213e10./1.0e10);
t47 = t32.*t33.*(2.6436969e7./2.5e9);
t48 = t8.*t28.*(2.30993127e8./5.0e9);
t49 = t15.*t22.*t24.*(2.30993127e8./5.0e9);
t50 = t8.*t19.*t20.*t23.*(2.1698418213e10./1.0e10);
t51 = t8.^2;
t52 = t7.*t23.*t51;
t53 = t15.^2;
t54 = t7.*t15.*t16.*t20;
t55 = t52+t54-t7.*t23.*t24.*t53;
t56 = t7.*t16.*t24;
t57 = t7.*t15.*t20.*t23;
t58 = t56+t57;
t59 = t8.*t19;
t60 = t7.*t15.*t16;
t61 = t59+t60;
t62 = t24.*t61;
t63 = t7.*t20.*t23;
t64 = t62+t63;
t65 = t15.*t20.*t61;
t66 = t65-t7.*t15.*t23.*t24;
t67 = t20.*t61;
t68 = t67-t7.*t23.*t24;
t69 = t15.*t19;
t70 = t69-t7.*t8.*t16;
t71 = t8.*t70;
t72 = t15.*t24.*t61;
t73 = t57+t71+t72;
torque= [0.0;t2.*(4.283174511e9./2.5e8)+t37+t38+t44+t46+t47+t48+t49+t50-t2.*t4.*(4.1664051e7./7.8125e7)-t7.*t15.*(3.09341673e8./1.0e10)-t7.*t39.*(2.934171e6./1.0e5)-t25.*t32.*(1.527243363e9./1.0e10)-t25.*t36.*(2.6436969e7./2.5e9)-t33.*t36.*(1.527243363e9./1.0e10)-t8.*t16.*t19.*(3.09341673e8./1.0e10)-t15.*t16.*t19.*(2.30993127e8./5.0e9)-t11.*t13.*t28.*(4.61382939e8./1.25e8)-t8.*t22.*t24.*(2.1698418213e10./1.0e10)-t15.*t19.*t20.*t23.*(2.30993127e8./5.0e9);-t37-t38-t44-t46-t47-t48-t49-t50+t2.*t4.*(4.1664051e7./7.8125e7)+t7.*t15.*(3.09341673e8./1.0e10)+t7.*t39.*(2.934171e6./1.0e5)+t25.*t32.*(1.527243363e9./1.0e10)+t25.*t36.*(2.6436969e7./2.5e9)+t33.*t36.*(1.527243363e9./1.0e10)+t8.*t16.*t19.*(3.09341673e8./1.0e10)+t15.*t16.*t19.*(2.30993127e8./5.0e9)+t11.*t13.*t28.*(4.61382939e8./1.25e8)+t8.*t22.*t24.*(2.1698418213e10./1.0e10)+t15.*t19.*t20.*t23.*(2.30993127e8./5.0e9);t40.*(-t7.*t8.*t16.*t20+t7.*t8.*t15.*t23+t7.*t8.*t15.*t23.*t24).*(-2.033613e6./1.0e5)+t25.*t55.*(2.6436969e7./2.5e9)-t25.*t58.*(1.527243363e9./1.0e10)+t33.*t55.*(1.527243363e9./1.0e10)+t33.*t58.*(2.6436969e7./2.5e9)+t7.*t8.*t23.*(3.09341673e8./1.0e10)+t7.*t13.*t23.*(4.61382939e8./1.25e8)+t7.*t15.*t23.*(2.30993127e8./5.0e9)-t7.*t23.*t51.*(2.30993127e8./5.0e9)+t7.*t8.*t16.*t20.*(2.1698418213e10./1.0e10)-t7.*t8.*t15.*t23.*(2.1698418213e10./1.0e10)-t7.*t15.*t16.*t20.*(2.30993127e8./5.0e9)+t7.*t23.*t24.*t53.*(2.30993127e8./5.0e9)-t7.*t8.*t15.*t23.*t24.*(2.1698418213e10./1.0e10);t40.*(t8.*t20.*t61-t7.*t8.*t23.*t24).*(2.033613e6./1.0e5)-t25.*t64.*(1.527243363e9./1.0e10)+t25.*t66.*(2.6436969e7./2.5e9)+t33.*t64.*(2.6436969e7./2.5e9)+t33.*t66.*(1.527243363e9./1.0e10)+t8.*t20.*t61.*(2.1698418213e10./1.0e10)-t15.*t20.*t61.*(2.30993127e8./5.0e9)-t7.*t8.*t23.*t24.*(2.1698418213e10./1.0e10)+t7.*t15.*t23.*t24.*(2.30993127e8./5.0e9);t25.*t68.*(2.6436969e7./2.5e9)-t25.*t73.*(1.527243363e9./1.0e10)+t33.*t68.*(1.527243363e9./1.0e10)+t33.*t73.*(2.6436969e7./2.5e9)];
% tau1=torque(1);
% tau2=torque(2);
% tau3=torque(3);
% tau4=torque(4);
% tau5=torque(5);
% tau6=torque(6);
